simulink model "model_testing_norml_modeslx_phanse"  (R2018b)
settings: Solver=ode3  StartTime=0.0  StopTime=2  RelTol=1e-3  EnableMultiTasking=on
PostLoadFcn:
  | Ts = 1/250;
undefined symbols (not defined in the file or in its folder): dev, Main, pwm_output0
libraries: simulink x4, px4Sensorslib x2, px4uORBlib x1, px4lib x1
Description:
  | PX4 PSP Example Model to show the RC Input Block working
  | 
  | Input RC Block Example
settings Model: Creator=skuznick  LastModifiedBy=Tejas Rajopadhye
settings SolverCC: PositivePriorityOrder=on
settings DataIOCC: LimitDataPoints=on  SaveFormat=Array  SignalLoggingSaveFormat=ModelDataLogs
settings OptimizationCC: DefaultParameterBehavior=Inlined  LifeSpan=1  MaxStackSize=64
settings DebuggingCC: SolverPrmCheckMsg=warning  MultiTaskDSMMsg=warning  MultiTaskCondExecSysMsg=none  AllowSymbolicDim=off  SFUnexpectedBacktrackingDiag=warning  SFNoUnconditionalDefaultTransitionDiag=warning  SFExecutionAtInitializationDiag=none
settings HardwareCC: ProdBitPerPointer=32  ProdBitPerSizeT=32  ProdBitPerPtrDiffT=32  ProdLargestAtomicInteger=Long  ProdLargestAtomicFloat=Double  ProdWordSize=32  ProdHWDeviceType=ARM Compatible->ARM Cortex
settings ModelReferenceCC: PropagateSignalLabelsOutOfModel=off
settings SFSimCC: SimUseLocalCustomCode=off  MATLABDynamicMemAlloc=off
settings RTWCC: SystemTargetFile=ert.tlc  HardwareBoard=Pixhawk PX4  TLCOptions="-aInlineSetEventsForThisBaseRateFcn=TLC_FALSE -aSuppressMultiTaskScheduler=TLC_FALSE    -aRateBasedStepFcn=0"  TemplateMakefile=ert_default_tmf  GenerateReport=on  RTWUseLocalCustomCode=off  Toolchain=Pixhawk Toolchain  BuildConfiguration=Faster Runs  IncludeHyperlinkInReport=on  LaunchReport=on  GenerateTraceReport=on  GenerateCodeMetricsReport=on
settings CodeAppCC: IgnoreCustomStorageClasses=off  StateflowObjectComments=on
settings ERTTargetCC: MultiwordLength=2048  ERTCustomFileTemplate=px4_codertarget_file_process.tlc  ConvertIfToSwitch=off  SuppressUnreachableDefaultCases=off
settings ConfigComp: CovMetricSettings=dw  CovHtmlReporting=on  CovSaveCumulativeToWorkspaceVar=on  CovSaveSingleToWorkspaceVar=on  CovExternalEMLEnable=off  CovSFcnEnable=off

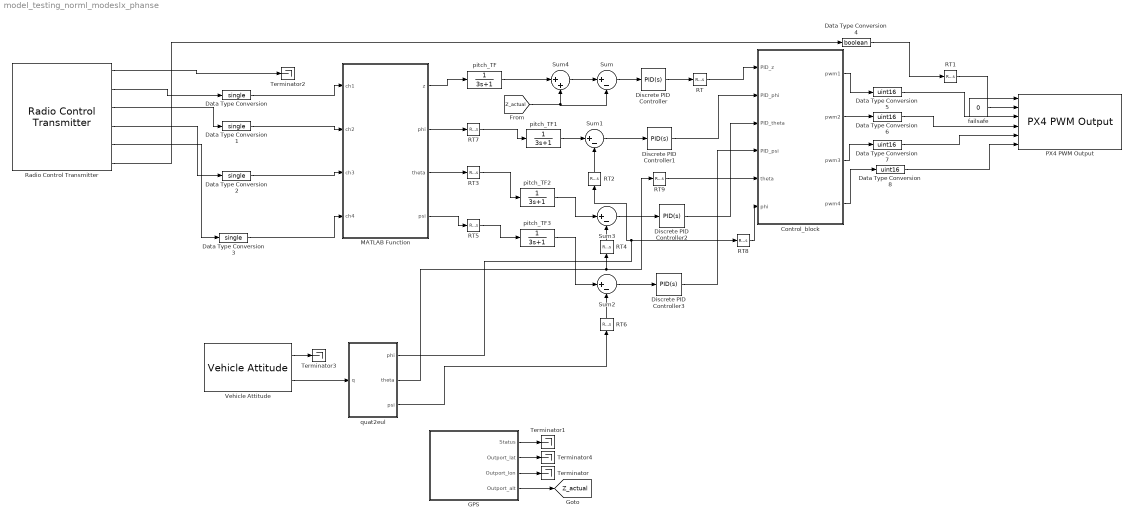
== system model_testing_norml_modeslx_phanse ==
  Control_block : MATLAB Function  TreatAsAtomicUnit=on
  Data Type Conversion{,1..3} (4 alike) : DataTypeConversion  OutDataTypeStr=single
  Data Type Conversion4 : DataTypeConversion  OutDataTypeStr=boolean
  Data Type Conversion{5..8} (4 alike) : DataTypeConversion  OutDataTypeStr=uint16
  Discrete PID Controller : simulink/Continuous/PID Controller  Controller=PID  Form=Parallel  TimeDomain=Continuous-time  SampleTime=-1  IntegratorMethod=Forward Euler  FilterMethod=Forward Euler  ControllerParametersSource=internal  P=20.5  I=2.5  D=55.5  UseFilter=on  N=100  TunerSelectOption=Transfer Function Based (PID Tuner App)  InitialConditionSource=internal  InitialConditionForIntegrator=0  InitialConditionForFilter=0  DifferentiatorICPrevScaledInput=0  ExternalReset=none  TrackingMode=off  Kt=1  LimitOutput=off  UpperSaturationLimit=inf  LowerSaturationLimit=-inf  LinearizeAsGain=off  AntiWindupMode=none  Kb=1  POutMin=[]  POutMax=[]  IOutMin=[]  IOutMax=[]  DOutMin=[]  DOutMax=[]  NOutMin=[]  NOutMax=[]  SumOutMin=[]  SumOutMax=[]  SaturationOutMin=[]  SaturationOutMax=[]  PParamMin=[]  PParamMax=[]  IParamMin=[]  IParamMax=[]  DParamMin=[]  DParamMax=[]  NParamMin=[]  NParamMax=[]  KbParamMin=[]  KbParamMax=[]  KtParamMin=[]  KtParamMax=[]  KbOutMin=[]  KbOutMax=[]  KtOutMin=[]  KtOutMax=[]  IntegratorOutMin=[]  IntegratorOutMax=[]  FilterOutMin=[]  FilterOutMax=[]  SumI1OutMin=[]  SumI1OutMax=[]  SumI2OutMin=[]  SumI2OutMax=[]  SumI3OutMin=[]  SumI3OutMax=[]  SumI4OutMin=[]  SumI4OutMax=[]  SumDOutMin=[]  SumDOutMax=[]  DifferentiatorOutMin=[]  DifferentiatorOutMax=[]  FilterDiffOutCoefMin=[]  FilterDiffOutCoefMax=[]  ReciprocalOutMin=[]  ReciprocalOutMax=[]  SumDenOutMin=[]  SumDenOutMax=[]  SumNumOutMin=[]  SumNumOutMax=[]  DivideOutMin=[]  DivideOutMax=[]  IntegratorContinuousStateAttributes=''  IntegratorStateMustResolveToSignalObject=off  IntegratorRTWStateStorageClass=Auto  FilterContinuousStateAttributes=''  FilterStateMustResolveToSignalObject=off  FilterRTWStateStorageClass=Auto  ParallelPVariant=InternalParameters  IdealPVariant=Disabled  IVariant=InternalParameters  DVariant=InternalParameters  IntegratorVariant=Continuous  SatVariant=Disabled  AWVariant=Passthrough  PCopyVariant=Disabled  TRVariant=Disabled  FdbkBlocksVariant=Forward  IdealPFdbkVariant=Disabled  SatFdbkVariant=Disabled  DerivativeFilterVariant=ContFilter  NVariant=InternalParameters  NCopyVariant=Disabled  FilterICVariant=InternalICsFilter  IntegratorICVariant=InternalICs  ExternalResetVariant=Disabled  TRSumVariant=Passthrough  SumFdbkVariant=Disabled  SumVariant=Sum_PID
  Discrete PID Controller1 : simulink/Continuous/PID Controller  Controller=PID  Form=Parallel  TimeDomain=Continuous-time  SampleTime=-1  IntegratorMethod=Forward Euler  FilterMethod=Forward Euler  ControllerParametersSource=internal  P=30  I=0.001  D=13  UseFilter=on  N=100  TunerSelectOption=Transfer Function Based (PID Tuner App)  InitialConditionSource=internal  InitialConditionForIntegrator=0  InitialConditionForFilter=0  DifferentiatorICPrevScaledInput=0  ExternalReset=none  TrackingMode=off  Kt=1  LimitOutput=off  UpperSaturationLimit=inf  LowerSaturationLimit=-inf  LinearizeAsGain=off  AntiWindupMode=none  Kb=1  POutMin=[]  POutMax=[]  IOutMin=[]  IOutMax=[]  DOutMin=[]  DOutMax=[]  NOutMin=[]  NOutMax=[]  SumOutMin=[]  SumOutMax=[]  SaturationOutMin=[]  SaturationOutMax=[]  PParamMin=[]  PParamMax=[]  IParamMin=[]  IParamMax=[]  DParamMin=[]  DParamMax=[]  NParamMin=[]  NParamMax=[]  KbParamMin=[]  KbParamMax=[]  KtParamMin=[]  KtParamMax=[]  KbOutMin=[]  KbOutMax=[]  KtOutMin=[]  KtOutMax=[]  IntegratorOutMin=[]  IntegratorOutMax=[]  FilterOutMin=[]  FilterOutMax=[]  SumI1OutMin=[]  SumI1OutMax=[]  SumI2OutMin=[]  SumI2OutMax=[]  SumI3OutMin=[]  SumI3OutMax=[]  SumI4OutMin=[]  SumI4OutMax=[]  SumDOutMin=[]  SumDOutMax=[]  DifferentiatorOutMin=[]  DifferentiatorOutMax=[]  FilterDiffOutCoefMin=[]  FilterDiffOutCoefMax=[]  ReciprocalOutMin=[]  ReciprocalOutMax=[]  SumDenOutMin=[]  SumDenOutMax=[]  SumNumOutMin=[]  SumNumOutMax=[]  DivideOutMin=[]  DivideOutMax=[]  IntegratorContinuousStateAttributes=''  IntegratorStateMustResolveToSignalObject=off  IntegratorRTWStateStorageClass=Auto  FilterContinuousStateAttributes=''  FilterStateMustResolveToSignalObject=off  FilterRTWStateStorageClass=Auto  ParallelPVariant=InternalParameters  IdealPVariant=Disabled  IVariant=InternalParameters  DVariant=InternalParameters  IntegratorVariant=Continuous  SatVariant=Disabled  AWVariant=Passthrough  PCopyVariant=Disabled  TRVariant=Disabled  FdbkBlocksVariant=Forward  IdealPFdbkVariant=Disabled  SatFdbkVariant=Disabled  DerivativeFilterVariant=ContFilter  NVariant=InternalParameters  NCopyVariant=Disabled  FilterICVariant=InternalICsFilter  IntegratorICVariant=InternalICs  ExternalResetVariant=Disabled  TRSumVariant=Passthrough  SumFdbkVariant=Disabled  SumVariant=Sum_PID
  Discrete PID Controller2 : simulink/Continuous/PID Controller  Controller=PID  Form=Parallel  TimeDomain=Continuous-time  SampleTime=-1  IntegratorMethod=Forward Euler  FilterMethod=Forward Euler  ControllerParametersSource=internal  P=11.05  I=0.01  D=10.05  UseFilter=on  N=100  TunerSelectOption=Transfer Function Based (PID Tuner App)  InitialConditionSource=internal  InitialConditionForIntegrator=0  InitialConditionForFilter=0  DifferentiatorICPrevScaledInput=0  ExternalReset=none  TrackingMode=off  Kt=1  LimitOutput=off  UpperSaturationLimit=inf  LowerSaturationLimit=-inf  LinearizeAsGain=off  AntiWindupMode=none  Kb=1  POutMin=[]  POutMax=[]  IOutMin=[]  IOutMax=[]  DOutMin=[]  DOutMax=[]  NOutMin=[]  NOutMax=[]  SumOutMin=[]  SumOutMax=[]  SaturationOutMin=[]  SaturationOutMax=[]  PParamMin=[]  PParamMax=[]  IParamMin=[]  IParamMax=[]  DParamMin=[]  DParamMax=[]  NParamMin=[]  NParamMax=[]  KbParamMin=[]  KbParamMax=[]  KtParamMin=[]  KtParamMax=[]  KbOutMin=[]  KbOutMax=[]  KtOutMin=[]  KtOutMax=[]  IntegratorOutMin=[]  IntegratorOutMax=[]  FilterOutMin=[]  FilterOutMax=[]  SumI1OutMin=[]  SumI1OutMax=[]  SumI2OutMin=[]  SumI2OutMax=[]  SumI3OutMin=[]  SumI3OutMax=[]  SumI4OutMin=[]  SumI4OutMax=[]  SumDOutMin=[]  SumDOutMax=[]  DifferentiatorOutMin=[]  DifferentiatorOutMax=[]  FilterDiffOutCoefMin=[]  FilterDiffOutCoefMax=[]  ReciprocalOutMin=[]  ReciprocalOutMax=[]  SumDenOutMin=[]  SumDenOutMax=[]  SumNumOutMin=[]  SumNumOutMax=[]  DivideOutMin=[]  DivideOutMax=[]  IntegratorContinuousStateAttributes=''  IntegratorStateMustResolveToSignalObject=off  IntegratorRTWStateStorageClass=Auto  FilterContinuousStateAttributes=''  FilterStateMustResolveToSignalObject=off  FilterRTWStateStorageClass=Auto  ParallelPVariant=InternalParameters  IdealPVariant=Disabled  IVariant=InternalParameters  DVariant=InternalParameters  IntegratorVariant=Continuous  SatVariant=Disabled  AWVariant=Passthrough  PCopyVariant=Disabled  TRVariant=Disabled  FdbkBlocksVariant=Forward  IdealPFdbkVariant=Disabled  SatFdbkVariant=Disabled  DerivativeFilterVariant=ContFilter  NVariant=InternalParameters  NCopyVariant=Disabled  FilterICVariant=InternalICsFilter  IntegratorICVariant=InternalICs  ExternalResetVariant=Disabled  TRSumVariant=Passthrough  SumFdbkVariant=Disabled  SumVariant=Sum_PID
  Discrete PID Controller3 : simulink/Continuous/PID Controller  Controller=PID  Form=Parallel  TimeDomain=Continuous-time  SampleTime=-1  IntegratorMethod=Forward Euler  FilterMethod=Forward Euler  ControllerParametersSource=internal  P=100  I=2  D=1  UseFilter=on  N=100  TunerSelectOption=Transfer Function Based (PID Tuner App)  InitialConditionSource=internal  InitialConditionForIntegrator=0  InitialConditionForFilter=0  DifferentiatorICPrevScaledInput=0  ExternalReset=none  TrackingMode=off  Kt=1  LimitOutput=off  UpperSaturationLimit=inf  LowerSaturationLimit=-inf  LinearizeAsGain=off  AntiWindupMode=none  Kb=1  POutMin=[]  POutMax=[]  IOutMin=[]  IOutMax=[]  DOutMin=[]  DOutMax=[]  NOutMin=[]  NOutMax=[]  SumOutMin=[]  SumOutMax=[]  SaturationOutMin=[]  SaturationOutMax=[]  PParamMin=[]  PParamMax=[]  IParamMin=[]  IParamMax=[]  DParamMin=[]  DParamMax=[]  NParamMin=[]  NParamMax=[]  KbParamMin=[]  KbParamMax=[]  KtParamMin=[]  KtParamMax=[]  KbOutMin=[]  KbOutMax=[]  KtOutMin=[]  KtOutMax=[]  IntegratorOutMin=[]  IntegratorOutMax=[]  FilterOutMin=[]  FilterOutMax=[]  SumI1OutMin=[]  SumI1OutMax=[]  SumI2OutMin=[]  SumI2OutMax=[]  SumI3OutMin=[]  SumI3OutMax=[]  SumI4OutMin=[]  SumI4OutMax=[]  SumDOutMin=[]  SumDOutMax=[]  DifferentiatorOutMin=[]  DifferentiatorOutMax=[]  FilterDiffOutCoefMin=[]  FilterDiffOutCoefMax=[]  ReciprocalOutMin=[]  ReciprocalOutMax=[]  SumDenOutMin=[]  SumDenOutMax=[]  SumNumOutMin=[]  SumNumOutMax=[]  DivideOutMin=[]  DivideOutMax=[]  IntegratorContinuousStateAttributes=''  IntegratorStateMustResolveToSignalObject=off  IntegratorRTWStateStorageClass=Auto  FilterContinuousStateAttributes=''  FilterStateMustResolveToSignalObject=off  FilterRTWStateStorageClass=Auto  ParallelPVariant=InternalParameters  IdealPVariant=Disabled  IVariant=InternalParameters  DVariant=InternalParameters  IntegratorVariant=Continuous  SatVariant=Disabled  AWVariant=Passthrough  PCopyVariant=Disabled  TRVariant=Disabled  FdbkBlocksVariant=Forward  IdealPFdbkVariant=Disabled  SatFdbkVariant=Disabled  DerivativeFilterVariant=ContFilter  NVariant=InternalParameters  NCopyVariant=Disabled  FilterICVariant=InternalICsFilter  IntegratorICVariant=InternalICs  ExternalResetVariant=Disabled  TRSumVariant=Passthrough  SumFdbkVariant=Disabled  SumVariant=Sum_PID
  GPS : Subsystem  mask(Vehicle GPS){lat=on, lon=on, alt=on, velocity=off, gpsfix=off, numsat=off, timestamp=off, BlockingMode=off, BlockTimeout=1e-3, sampleTime=1/250}
      mask prompts: lat "Latitude (1e-7 degress)"; lon "Longitude (1e-7 degress)"; alt "Altitude (mm)"; velocity "Velocity (m/s)"; gpsfix "GPS Fix Type"; numsat "Number of satellites"; timestamp "Timestamp (microseconds)"; BlockingMode "px4:blockmask:SubscriberBlockingMode"; BlockTimeout "px4:blockmask:SubscriberBlockingModeTimeout"; sampleTime "px4:blockmask:SampleTimePrompt"
      mask help:
      | Read Vehicle GPS values using 'vehicle_gps_position' uORB topic.  Select the required GPS values from the list below.
      |
      | Status is a boolean value indicating whether a GPS values was received during the previous time step. When Status is 0, GPS values holds the newly-received message. When Status is 1, GPS values holds the last received message.
      | The Latitude, Longitude and Altitude are scalar values of datatype int32 and Velocity is of datatype single. GPS Fix Type and Number of satellites are scalars of datatype uint8.
      | The Timestamp is the absolute time value when the last message was recieved and is a scalar of datatype uint64.
      mask init:
      | % List of signals required as output
      | signal_names = {'<lat>','<lon>','<alt>','<vel_m_s>','<fix_type>',...
      |                         '<satellites_used>','<timestamp>'};
      | %Output port names to display in the mask
      | output_port_names = {'Latitude','Longitude','Altitude',...
      |                         'Velocity','Fix Type','Num Satellites',...
      |                         'Timestamp'};
      | %Fullpath to the mask image
      | mask_image = [];
      | px4.internal.block.CommonuORBTopicMask.commonMaskCallback(gcb,signal_names,output_port_names,mask_image);
      mask Help: eval('codertarget.internal.helpView(''px4'',''px4vehiclegps'')');
      mask TypeOptions BlockingMode: PX4 uORB Read/BlockingMode
      mask Callback BlockingMode: px4.internal.block.CommonuORBTopicMask.blockingModeCallback(gcb);
      mask TypeOptions BlockTimeout: PX4 uORB Read/BlockTimeout
      mask TypeOptions sampleTime: PX4 uORB Read/sampleTime
      mask DialogControl Container6 Prompt: Main
      mask DialogControl Container11 Prompt: Advanced
      mask DialogControl BlockingMode Prompt: Wait until data received
      mask DialogControl BlockTimeout Prompt: Timeout in seconds:
      mask DialogControl sampleTime Prompt: Sample time (-1 for inherited):
      mask Display:
      | color('blue');
      | text(0.25, 0.9, 'PX4', 'horizontalAlignment', 'right');
      | color('black');
      | text(0.5, 0.5, get_param(gcb,'MaskType'), 'horizontalAlignment', 'center');
      | port_label('output',1,'Status');
      | port_label('output',2,'Latitude');
      | port_label('output',3,'Longitude');
      | port_label('output',4,'Altitude');
  MATLAB Function : MATLAB Function  TreatAsAtomicUnit=on
  PX4 PWM Output : px4lib/PX4 PWM Output  pwmDevice=Main (/dev/pwm_output0)  pwmChannel1_=on  pwmChannel2_=on  pwmChannel3_=on  pwmChannel4_=on  pwmChannel5_=off  pwmChannel6_=off  pwmChannel7_=off  pwmChannel8_=off  forceTerminateFailsafe=off  outputErrorStatus=off
      settings: SourceProductName=Embedded Coder Support Package for PX4 Autopilots  SourceProductBaseCode=PX4AUTOPILOTS
  RT{,1..9} (10 alike) : RateTransition  OutPortSampleTime=0.002
  Radio Control Transmitter : px4Sensorslib/Radio Control Transmitter  channel1=on  channel2=on  channel3=on  channel4=on  channel5=on  channel6=off  channel7=off  channel8=off  channel_count=off  rssi=off  rc_input_source=off  timestamp_last_signal=off  time_stamp=off  sampleTime=1/250  BlockingMode=off  BlockTimeout=5
      settings: SourceProductName=Embedded Coder Support Package for PX4 Autopilots
  Sum{,1..3} (4 alike) : Sum  Inputs=|+-
  Sum4 : Sum  Inputs=|++
  Terminator{,1..4} (5 alike) : Terminator
  Vehicle Attitude : px4Sensorslib/Vehicle Attitude  rollRate=off  pitchRate=off  yawRate=off  quaternion=on  uorbTimeStamp=off  BlockingMode=off  BlockTimeout=0.001  sampleTime=1/250
      settings: SourceProductName=Embedded Coder Support Package for PX4 Autopilots
  failsafe : Constant  Value=0  OutDataTypeStr=boolean  SampleTime=0.01
  pitch_TF{,1..3} (4 alike) : TransferFcn  Denominator=[3 1]
  quat2eul : MATLAB Function  TreatAsAtomicUnit=on
  tag scope: Z_actual=global
  wires:
  Sum2/1 -> Discrete PID Controller3/1
  Discrete PID Controller2/1 -> Control_block/3(PID_theta)
  Discrete PID Controller1/1 -> Control_block/2(PID_phi)
  Data Type Conversion6/1 -> PX4 PWM Output/4
  Data Type Conversion7/1 -> PX4 PWM Output/5
  Sum3/1 -> Discrete PID Controller2/1
  RT6/1 -> Sum2/2
  Control_block/2(pwm2) -> Data Type Conversion6/1
  Discrete PID Controller/1 -> RT/1
  Data Type Conversion5/1 -> PX4 PWM Output/3
  GPS/3(Outport_lon) -> Terminator/1
  Radio Control Transmitter/6 -> Data Type Conversion4/1
  Data Type Conversion4/1 -> RT1/1
  RT4/1 -> Sum3/2
  Data Type Conversion3/1 -> MATLAB Function/4(ch4)
  Radio Control Transmitter/4 -> Data Type Conversion2/1
  Data Type Conversion/1 -> MATLAB Function/1(ch1)
  Radio Control Transmitter/5 -> Data Type Conversion3/1
  Data Type Conversion8/1 -> PX4 PWM Output/6
  Radio Control Transmitter/3 -> Data Type Conversion1/1
  quat2eul/1(phi) -> RT2/1, RT8/1
  Data Type Conversion1/1 -> MATLAB Function/2(ch2)
  Control_block/3(pwm3) -> Data Type Conversion7/1
  Control_block/1(pwm1) -> Data Type Conversion5/1
  quat2eul/3(psi) -> RT6/1
  MATLAB Function/2(phi) -> RT7/1
  MATLAB Function/4(psi) -> RT5/1
  Sum1/1 -> Discrete PID Controller1/1
  Data Type Conversion2/1 -> MATLAB Function/3(ch3)
  Vehicle Attitude/2 -> quat2eul/1(q)
  Sum/1 -> Discrete PID Controller/1
  Radio Control Transmitter/2 -> Data Type Conversion/1
  MATLAB Function/3(theta) -> RT3/1
  Control_block/4(pwm4) -> Data Type Conversion8/1
  quat2eul/2(theta) -> RT4/1, RT9/1
  RT/1 -> Control_block/1(PID_z)
  RT1/1 -> PX4 PWM Output/1
  Discrete PID Controller3/1 -> Control_block/4(PID_psi)
  RT2/1 -> Sum1/2
  RT8/1 -> Control_block/6(phi)
  RT9/1 -> Control_block/5(theta)
  MATLAB Function/1(z) -> pitch_TF/1
  pitch_TF1/1 -> Sum1/1
  RT7/1 -> pitch_TF1/1
  pitch_TF2/1 -> Sum3/1
  RT3/1 -> pitch_TF2/1
  pitch_TF3/1 -> Sum2/1
  RT5/1 -> pitch_TF3/1
  Radio Control Transmitter/1 -> Terminator2/1
  GPS/4(Outport_alt) -> [Z_actual]
  pitch_TF/1 -> Sum4/1
  Sum4/1 -> Sum/1
  [Z_actual] -> Sum4/2, Sum/2
  Vehicle Attitude/1 -> Terminator3/1
  GPS/1(Status) -> Terminator1/1
  GPS/2(Outport_lat) -> Terminator4/1
  failsafe/1 -> PX4 PWM Output/2

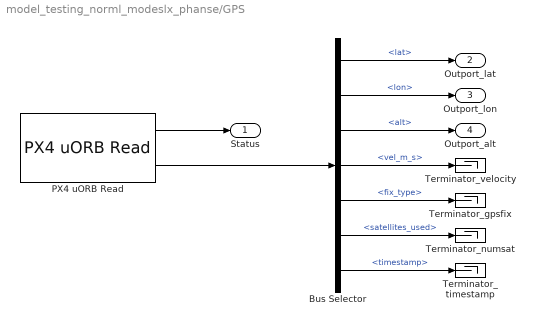
== system model_testing_norml_modeslx_phanse/GPS ==
  Bus Selector : BusSelector  OutputSignals=lat,lon,alt,vel_m_s,fix_type,satellites_used,timestamp
  PX4 uORB Read : px4uORBlib/PX4 uORB Read  uORBTopic=vehicle_gps_position  sampleTime=sampleTime  BlockingMode=off  BlockTimeout=BlockTimeout
      settings: SourceProductName=Embedded Coder Support Package for PX4 Autopilots
  Terminator_gpsfix : Terminator
  Terminator_numsat : Terminator
  Terminator_timestamp : Terminator
  Terminator_velocity : Terminator
  Status : Outport
  Outport_lat : Outport  Port=2
  Outport_lon : Outport  Port=3
  Outport_alt : Outport  Port=4
  wires:
  Bus Selector/2 -> Outport_lon/1  "<lon>"
  Bus Selector/1 -> Outport_lat/1  "<lat>"
  Bus Selector/7 -> Terminator_timestamp/1  "<timestamp>"
  Bus Selector/6 -> Terminator_numsat/1  "<satellites_used>"
  Bus Selector/5 -> Terminator_gpsfix/1  "<fix_type>"
  Bus Selector/4 -> Terminator_velocity/1  "<vel_m_s>"
  Bus Selector/3 -> Outport_alt/1  "<alt>"
  PX4 uORB Read/1 -> Status/1
  PX4 uORB Read/2 -> Bus Selector/1

== matlab function model_testing_norml_modeslx_phanse/Control_block ==
  data: PID_z input; pwm1 output; PID_phi input; PID_theta input; PID_psi input; pwm2 output; pwm3 output; pwm4 output; theta input; phi input
function [pwm1, pwm2, pwm3, pwm4] = Control_block(PID_z, PID_phi, PID_theta, PID_psi, theta, phi)
%#codegen


Ixx = single(0.047);
Iyy = single(0.047);
Izz = single(0.094);

g = 9.81;
l = 0.225;

ct = 0.0984;    % Values from doc
cm = 0.00679;   % Values from doc

%Complete the instrutions
T = 0.93*g + PID_z /(cos(theta)*cos(phi)); %U4 This is a more logical way of writing the torque term
tauphi = PID_phi*Ixx;
tautheta = PID_theta*Iyy;
taupsi = PID_psi*Izz;

% w1 w2 .... Made changes in the signs according to our calculations and
% model... make sure you do the right connections on the setup

w1 = T/(4*ct) - tautheta/(2*ct*l) - taupsi/(4*cm);
w2 = T/(4*ct) - tauphi/(2*ct*l) + taupsi/(4*cm);
w3 = T/(4*ct) + tautheta/(2*ct*l) - taupsi/(4*cm);
w4 = T/(4*ct) + tauphi/(2*ct*l) + taupsi/(4*cm);


% Taking sqrt of all omega's
w1 = sqrt(w1);
w2 = sqrt(w2);
w3 = sqrt(w3);
w4 = sqrt(w4);


% convert omegas to Pwm values and give the output to pwm block
% From this answer that i got from net about working of ESC's (https://electronics.stackexchange.com/questions/42616/how-to-use-an-esc)
% 100 % Pwm --> 2.0ms (@50hz) --> maxSpeed (11000rpm)
% Using that logic 2,5ms*Xrpm/ 11000rpm will give us the required PWM

pwm1 = (w1*2.0e-3)/11000;
pwm2 = (w2*2.0e-3)/11000;
pwm3 = (w3*2.0e-3)/11000;
pwm4 = (w4*2.0e-3)/11000;

== matlab function model_testing_norml_modeslx_phanse/MATLAB Function ==
  data: ch1 input; z output; ch2 input; ch3 input; ch4 input; phi output; theta output; psi output
function [z, phi, theta, psi] = convertto(ch1, ch2, ch3, ch4)
%#codegen

z = ch1 - 1000;
theta = ch2 - 1000;
psi =  ch3 - 1000;
phi = ch4 - 1000;

== matlab function model_testing_norml_modeslx_phanse/quat2eul ==
  data: q input; phi output; theta output; psi output
function [phi,theta,psi] = quat2eul(q)
% Conversion from Quaternion to Euler angles based on the PX4 Firmware
% v1.6.5 release.
% 
% Quaternion -> DCM -> Euler Angles
% INPUT:
%   q: Quaternion vector of the format: (a + bi + cj + dk)
% OUTPUT:
%   [phi,theta,psi]: Euler angles in radians.
% 
 
    a = q(1);
    b = q(2);
    c = q(3);
    d = q(4);

    aSq = a*a;
    bSq = b*b;
    cSq = c*c;
    dSq = d*d;

    d_pi2 = pi/2;

    % quaternion_to_dcm
    dcm00 = aSq + bSq - cSq - dSq;
    % dcm01 = 2*(b*c - a*d);
    dcm02 = 2*(a*c + b*d);
    dcm10 = 2*(b*c + a*d);
    % dcm11 = aSq - bSq + cSq - dSq;
    dcm12 = 2*(c*d - a*b);
    dcm20 = 2*(b*d - a*c);
    dcm21 = 2*(a*b + c*d);
    dcm22 = aSq - bSq - cSq + dSq;

    % dcm_to_euler
    theta = asin(-dcm20);
    if abs(theta - d_pi2) < 1.0e-3
        phi = single(0.0);
        psi = atan2(dcm12, dcm02);
    elseif abs(theta + d_pi2) < 1.0e-3
        phi = single(0.0);
        psi = atan2(-dcm12, -dcm02);
    else
        phi = atan2(dcm21, dcm22);
        psi = atan2(dcm10, dcm00);
    end

end
